simulink model "PendulumModel"  (R2018b)
settings: Solver=VariableStepAuto  StartTime=0.0  StopTime=10.0  RelTol=1e-3
settings Model: Creator=Yahya  LastModifiedBy=Yahya

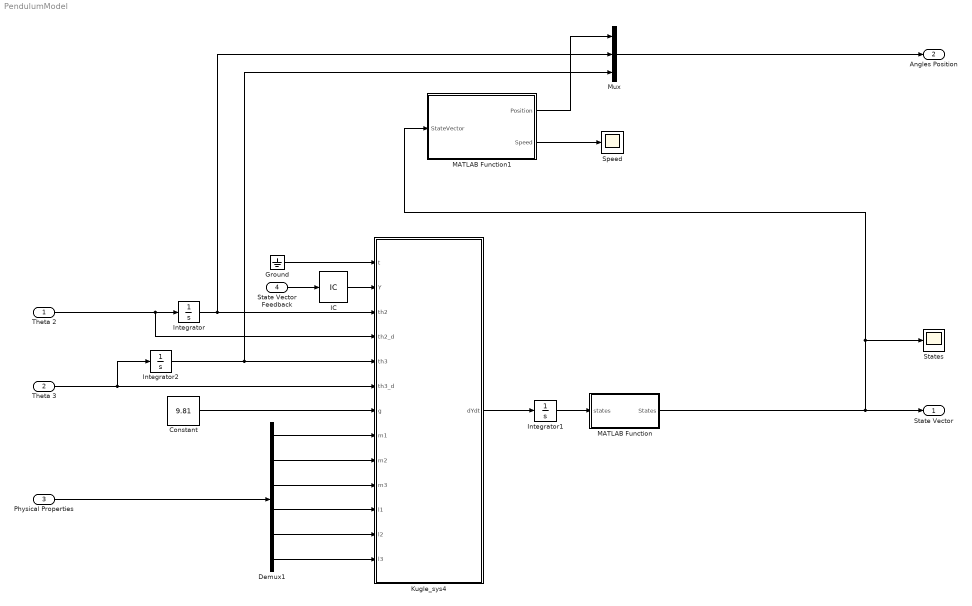
== system PendulumModel ==
  Theta 2 : Inport  PortDimensions=1
  Theta 3 : Inport  Port=2  PortDimensions=1
  Physical Properties : Inport  Port=3
  State Vector Feedback : Inport  Port=4  PortDimensions=2
  Constant : Constant  Value=9.81
  Demux1 : Demux  Outputs=6
  Ground : Ground
  IC : InitialCondition  Value=[0 0]
  Integrator : Integrator
  Integrator1 : Integrator  InitialCondition=[0 0]*pi/180
  Integrator2 : Integrator
  Kugle_sys4 : MATLAB Function  TreatAsAtomicUnit=on
  MATLAB Function : MATLAB Function  TreatAsAtomicUnit=on
  MATLAB Function1 : MATLAB Function  TreatAsAtomicUnit=on
  Mux : Mux  Inputs=3
  Speed : Scope
  States : Scope
  State Vector : Outport  PortDimensions=2
  Angles Position : Outport  Port=2
  wires:
  Demux1/2 -> Kugle_sys4/9(m2)
  Constant/1 -> Kugle_sys4/7(g)
  MATLAB Function/1(States) -> MATLAB Function1/1(StateVector), States/1, State Vector/1
  Ground/1 -> Kugle_sys4/1(t)
  Demux1/4 -> Kugle_sys4/11(l1)
  Demux1/5 -> Kugle_sys4/12(l2)
  Demux1/6 -> Kugle_sys4/13(l3)
  Integrator2/1 -> Mux/3, Kugle_sys4/5(th3)
  Integrator1/1 -> MATLAB Function/1(states)
  Integrator/1 -> Mux/2, Kugle_sys4/3(th2)
  MATLAB Function1/1(Position) -> Mux/1
  Demux1/3 -> Kugle_sys4/10(m3)
  Demux1/1 -> Kugle_sys4/8(m1)
  MATLAB Function1/2(Speed) -> Speed/1
  Mux/1 -> Angles Position/1
  Physical Properties/1 -> Demux1/1
  Theta 2/1 -> Kugle_sys4/4(th2_d), Integrator/1
  Theta 3/1 -> Integrator2/1, Kugle_sys4/6(th3_d)
  Kugle_sys4/1(dYdt) -> Integrator1/1
  State Vector Feedback/1 -> IC/1
  IC/1 -> Kugle_sys4/2(Y)

== matlab function PendulumModel/Kugle_sys4 ==
  data: t input; dYdt output; Y input; th2 input; th2_d input; th3 input; th3_d input; g input; m1 input; m2 input; m3 input; l1 input; l2 input; l3 input
function dYdt = Kugle_sys4(t,Y,th2,th2_d,th3,th3_d,g,m1,m2,m3,l1,l2,l3)
%#codegen

%    This function was generated by the Symbolic Math Toolbox version 8.2.
%    22-Apr-2019 11:19:29

t2 = Y(1);
t3 = t2+th2;
t4 = sin(t3);
t5 = sin(t2);
t6 = l1.^2;
t7 = l2.^2;
t8 = cos(th2);
dYdt = [Y(2);((g.*l1.*m1.*t5+g.*l1.*m2.*t5.*2.0+g.*l2.*m2.*t4+g.*l1.*m3.*t5.*2.0+g.*l2.*m3.*t4.*2.0+g.*l3.*m3.*sin(t2+th2+th3)).*(3.0./2.0))./(m1.*t6+m2.*t6.*3.0+m2.*t7+m3.*t6.*3.0+m3.*t7.*3.0+l3.^2.*m3+l1.*l2.*m2.*t8.*3.0+l1.*l2.*m3.*t8.*6.0+l1.*l3.*m3.*cos(th2+th3).*3.0+l2.*l3.*m3.*cos(th3).*3.0)];

== matlab function PendulumModel/MATLAB Function ==
  data: states input; States output
function States = angleLimit(states)

vec = [0 0];

vec(2) = states(2);

vec(1) = angError(states(1));

States = vec;

== matlab function PendulumModel/MATLAB Function1 ==
  data: StateVector input; Position output; Speed output
function [Position, Speed] = StateSeparator(StateVector)

Position = StateVector(1);

Speed = StateVector(2);
